simulink model "tuoyuan"  (R2023b)
settings: Solver=FixedStepAuto  StartTime=0.0  StopTime=50  FixedStep=1e-3  RelTol=1e-3
undefined symbols (not defined in the file or in its folder): w
settings Model: Creator=asus  LastModifiedBy=asus

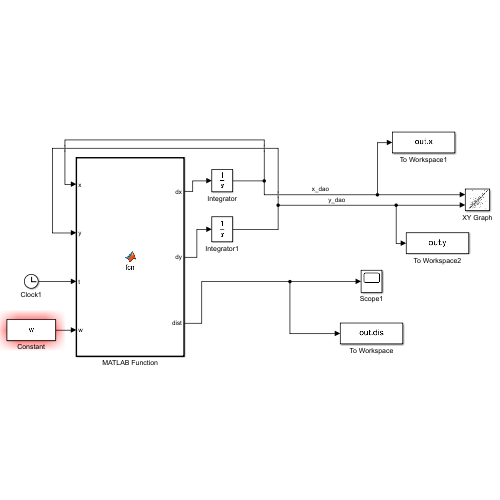
[thumbnail: Simulink's stored preview of the top-level diagram]
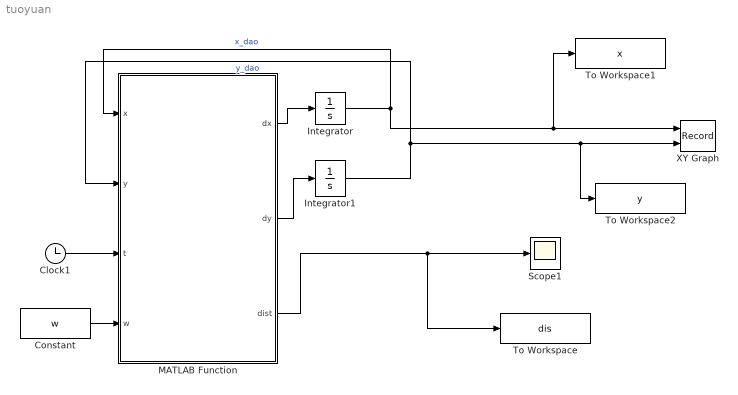
== system tuoyuan ==
  Clock1 : Clock
  Constant : Constant  Value=w
  Integrator : Integrator
  Integrator1 : Integrator
  MATLAB Function : MATLAB Function  TreatAsAtomicUnit=on
  Scope1 : Scope
  To Workspace : ToWorkspace  VariableName=dis  SaveFormat=Timeseries  SampleTime=-1
  To Workspace1 : ToWorkspace  VariableName=x  SaveFormat=Timeseries  SampleTime=-1
  To Workspace2 : ToWorkspace  VariableName=y  SaveFormat=Timeseries  SampleTime=-1
  XY Graph : Record  FileSettingsInternal="{\"entries\":[{\"content\":{\"excelSettings\":{\"content\":{},\"type\":\"Streamout.ExcelSettings\"}},\"type\":\"Streamout.FileSettingStorage\",\"uuid\":\"\"}],\"packageUris\":[\"http:\\/\\/schema.mathworks.com\\/mf0\\/streamout_blocks\\/R2020a\"],\"version\":\"1.0\"}"  Layout=[1 1]  SignalsInternal="{\"entries\":[{\"content\":{\"signals\":[{\"content\":{\"blockPath\":[],\"dimensions\":[1],\"domain\":\"\",\"lineColor\":\"#a2142f\",\"plots\":[1],\"port\":1,\"sid\":[\"\"],\"signalID\":6282,\"signalName\":\"x_dao\"},\"type\":\"RecordBlkView.Signal\",\"uuid\":\"\"},{\"content\":{\"blockPath\":[],\"dimensions\":[1],\"domain\":\"\",\"lineColor\":\"#139fff\",\"plots\":[1],\"port\":2,\"sid\":[\"\"],\"signalID\":6286,\"signalName\":\"y_dao\"},\"type\":\"RecordBlkView.Signal\",\"uuid\":\"\"}]},\"type\":\"RecordBlkView.InputSignals\",\"uuid\":\"\"}],\"packageUris\":[\"http:\\/\\/schema.mathworks.com\\/mf0\\/streamout_blocks\\/R2020a\"],\"version\":\"1.0\"}"  VisualizationBindings="{\"xyplotplugin\":{\"info\":[{\"series\":[{\"bindingParametersList\":[{\"parameter\":\"X-Axis\",\"signalID\":6282,\"signalName\":\"x_dao\"},{\"parameter\":\"Y-Axis\",\"signalID\":6286,\"signalName\":\"y_dao\"}],\"seriesID\":14509}],\"subplotID\":1}]}}"  CompatibilityTag=XY
  wires:
  MATLAB Function/1(dx) -> Integrator/1
  Integrator/1 -> To Workspace1/1, XY Graph/1, MATLAB Function/1(x)  "x_dao"
  Integrator1/1 -> To Workspace2/1, XY Graph/2, MATLAB Function/2(y)  "y_dao"
  MATLAB Function/2(dy) -> Integrator1/1
  Clock1/1 -> MATLAB Function/3(t)
  Constant/1 -> MATLAB Function/4(w)
  MATLAB Function/3(dist) -> To Workspace/1, Scope1/1

== matlab function tuoyuan/MATLAB Function ==
  data: x input; dx output; y input; t input; dy output; dist output; w input
function [dx,dy,dist] = fcn(x,y,t,w)
x_fei = 10 + 20*cos(t);
y_fei = 20 + 5*sin(t);
dist = sqrt( (x_fei - x)^2 + (y_fei - y)^2 );
dx = w * (x_fei - x) / dist;
dy = w * (y_fei - y) / dist;
